simulink model "model_model_Harness1"  (R2023a)
settings: Solver=VariableStepAuto  StartTime=0.0  StopTime=1  RelTol=1e-3
settings Model: Creator=diontep  LastModifiedBy=diontep

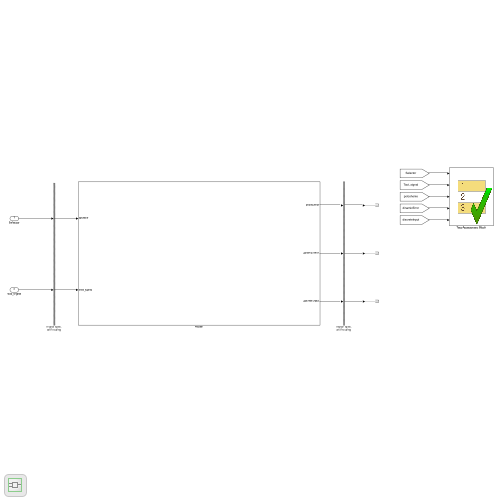
[thumbnail: Simulink's stored preview of the top-level diagram]
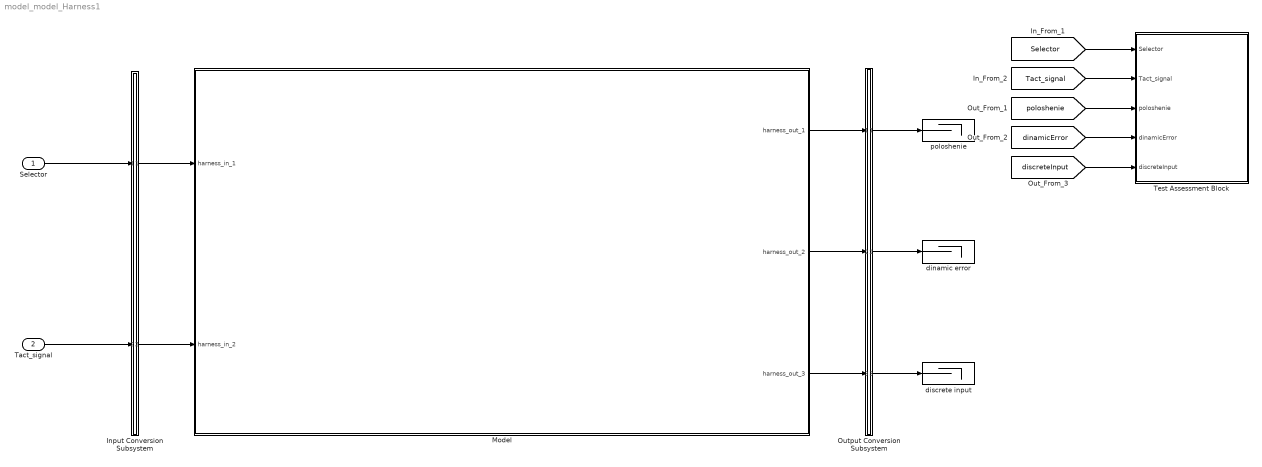
== system model_model_Harness1 ==
  Selector : Inport  OutDataTypeStr=double  PortDimensions=[1]  SampleTime=[-1, 0]
  Tact_signal : Inport  Port=2  OutDataTypeStr=double  PortDimensions=[1]  SampleTime=[0, 1]
  Input Conversion Subsystem : Subsystem  Tag=__SLT_ICS__  Description=|
      | Signal spec.
      | and routing
      settings: AttributesFormatString=%<Description>
  Model : Subsystem  Tag=__SL_testing_harness_stub_
  Output Conversion Subsystem : Subsystem  Tag=__SLT_OCS__  Description=|
      | Signal spec.
      | and routing
      settings: AttributesFormatString=%<Description>
  Test Assessment Block : Test Sequence  Tag=__SLT_ASMT__  TreatAsAtomicUnit=on
  dinamic error : Terminator
  discrete input : Terminator
  poloshenie : Terminator
  wires:
  [Selector] -> Test Assessment Block/1(Selector)
  [Tact_signal] -> Test Assessment Block/2(Tact_signal)
  [poloshenie] -> Test Assessment Block/3(poloshenie)
  [dinamicError] -> Test Assessment Block/4(dinamicError)
  [discreteInput] -> Test Assessment Block/5(discreteInput)
  Selector/1 -> Input Conversion Subsystem/1(Inport_1)
  Tact_signal/1 -> Input Conversion Subsystem/2(Inport_2)
  Output Conversion Subsystem/1(Outport_1) -> poloshenie/1
  Output Conversion Subsystem/2(Outport_2) -> dinamic error/1
  Output Conversion Subsystem/3(Outport_3) -> discrete input/1
  Input Conversion Subsystem/1(Outport_1) -> Model/1(harness_in_1)
  Input Conversion Subsystem/2(Outport_2) -> Model/2(harness_in_2)
  Model/1(harness_out_1) -> Output Conversion Subsystem/1(Inport_1)
  Model/2(harness_out_2) -> Output Conversion Subsystem/2(Inport_2)
  Model/3(harness_out_3) -> Output Conversion Subsystem/3(Inport_3)

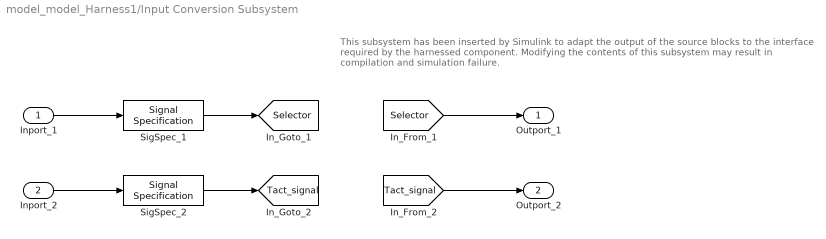
== system model_model_Harness1/Input Conversion Subsystem ==
  note: This subsystem has been inserted by Simulink to adapt the output of the source blocks to the interface required by the harnessed component.
      |  Modifying the contents of this subsystem may result in compilation and simulation failure.
  Inport_1 : Inport
  Inport_2 : Inport  Port=2
  SigSpec_1 : SignalSpecification  OutDataTypeStr=double  Dimensions=[1]  SampleTime=[-1, 0]
  SigSpec_2 : SignalSpecification  OutDataTypeStr=double  Dimensions=[1]  SampleTime=[0, 1]
  Outport_1 : Outport
  Outport_2 : Outport  Port=2
  tag scope: Selector=global, Tact_signal=global
  wires:
  [Selector] -> Outport_1/1
  SigSpec_1/1 -> [Selector]
  Inport_1/1 -> SigSpec_1/1
  [Tact_signal] -> Outport_2/1
  SigSpec_2/1 -> [Tact_signal]
  Inport_2/1 -> SigSpec_2/1

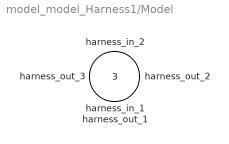
== system model_model_Harness1/Model ==
  harness_in_1 : Inport
  harness_in_2 : Inport  Port=2
  harness_out_1 : Outport
  harness_out_2 : Outport  Port=2
  harness_out_3 : Outport  Port=3

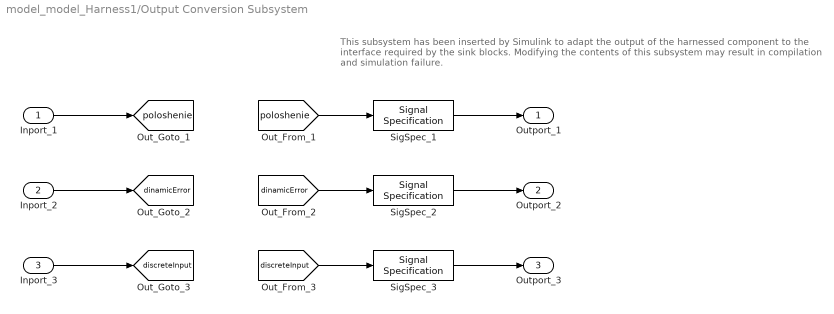
== system model_model_Harness1/Output Conversion Subsystem ==
  note: This subsystem has been inserted by Simulink to adapt the output of the harnessed component to the interface required by the sink blocks.
      |  Modifying the contents of this subsystem may result in compilation and simulation failure.
  Inport_1 : Inport
  Inport_2 : Inport  Port=2
  Inport_3 : Inport  Port=3
  SigSpec_1 : SignalSpecification  OutDataTypeStr=double  Dimensions=[1]
  SigSpec_2 : SignalSpecification  OutDataTypeStr=double  Dimensions=[1]
  SigSpec_3 : SignalSpecification  OutDataTypeStr=double  Dimensions=[1]
  Outport_1 : Outport
  Outport_2 : Outport  Port=2
  Outport_3 : Outport  Port=3
  tag scope: dinamicError=global, discreteInput=global, poloshenie=global
  wires:
  Inport_1/1 -> [poloshenie]
  [poloshenie] -> SigSpec_1/1
  SigSpec_1/1 -> Outport_1/1
  Inport_2/1 -> [dinamicError]
  [dinamicError] -> SigSpec_2/1
  SigSpec_2/1 -> Outport_2/1
  Inport_3/1 -> [discreteInput]
  [discreteInput] -> SigSpec_3/1
  SigSpec_3/1 -> Outport_3/1

== stateflow chart model_model_Harness1/Test Assessment Block ==
  state Run
    state step_1_1
    state step_1_2
    (default) -> (junction 22)
    Run -> (junction 22)
    (junction 22) -> (junction 23) [order 1] : [t < 5
        | ]
    (junction 23) -> step_1_1 [order 1] : [~in(Run.step_1_1)]
    (junction 23) -> (junction 26) [order 2]
    (junction 31) -> (junction 32)
    (junction 32) -> step_1_2 [order 1] : [~in(Run.step_1_2)]
    (junction 32) -> (junction 35) [order 2]
    (junction 22) -> (junction 31) [order 2]
  (default) -> Run
  data: Selector input double size=[1]; Tact_signal input double size=[1]; poloshenie input double size=[1]; dinamicError input double size=[1]; discreteInput input double size=[1]
